simulink model "MPTC"  (R2023b)
settings: Solver=FixedStepDiscrete  StartTime=0.0  StopTime=0.4  RelTol=1e-3
model workspace (MAT data in the model file):
  Ts = 0.025
undefined symbols (not defined in the file): DiscIntNeverNeededParam
libraries: spsDCVoltageSourceLib x1, spsGroundLib x1, spsPermanentMagnetSynchronousMachineLib x1, slpidlib x1, spsThreePhaseVIMeasurementLib x1, spsUniversalBridgeLib x1, sps_lib x1
settings Model: Creator=rainy  LastModifiedBy=rainy

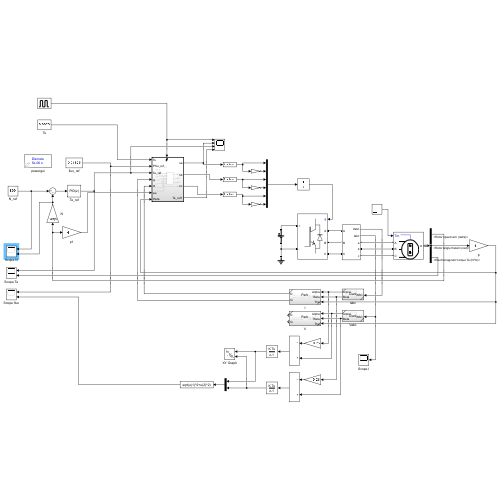
[thumbnail: Simulink's stored preview of the top-level diagram]
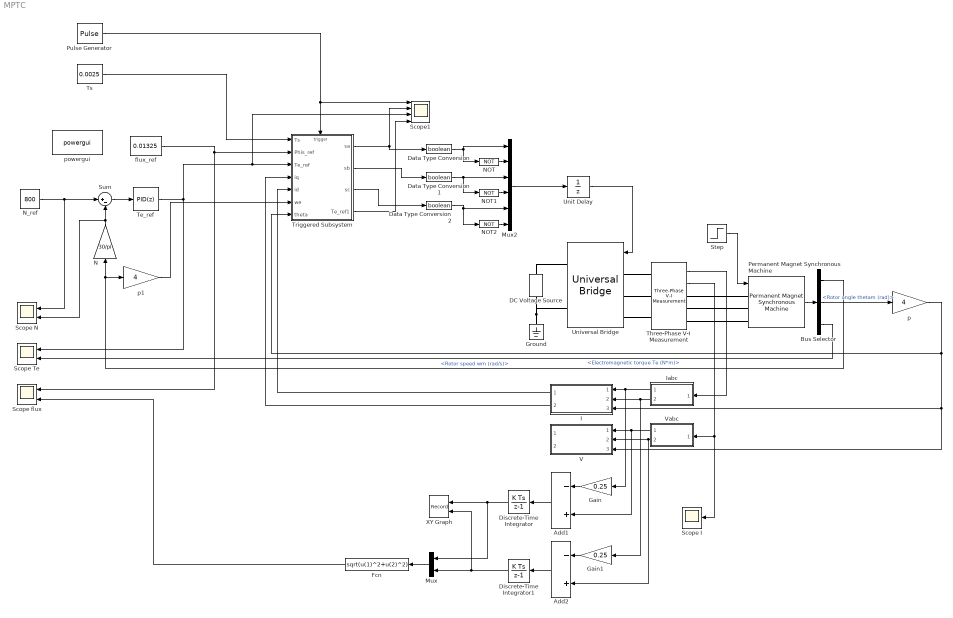
== system MPTC ==
  Add1 : Sum  Inputs=-+
  Add2 : Sum  Inputs=-+
  Bus Selector : BusSelector  OutputSignals=Rotor speed wm (rad/s),Rotor angle thetam (rad),Electromagnetic torque Te (N*m)
  DC Voltage Source : spsDCVoltageSourceLib/DC Voltage Source  Amplitude=24  Measurements=Voltage
  Data Type Conversion : DataTypeConversion  OutDataTypeStr=boolean  SaturateOnIntegerOverflow=off  RndMeth=Floor
  Data Type Conversion1 : DataTypeConversion  OutDataTypeStr=boolean  SaturateOnIntegerOverflow=off  RndMeth=Floor
  Data Type Conversion2 : DataTypeConversion  OutDataTypeStr=boolean  SaturateOnIntegerOverflow=off  RndMeth=Floor
  Discrete-Time Integrator : DiscreteIntegrator  SampleTime=-1  ICPrevOutput=DiscIntNeverNeededParam  ICPrevScaledInput=DiscIntNeverNeededParam
  Discrete-Time Integrator1 : DiscreteIntegrator  SampleTime=-1  ICPrevOutput=DiscIntNeverNeededParam  ICPrevScaledInput=DiscIntNeverNeededParam
  Fcn : Fcn  Expr=sqrt(u(1)^2+u(2)^2)
  Gain : Gain  Gain=0.25
  Gain1 : Gain  Gain=0.25
  Ground : spsGroundLib/Ground  LConnTagsString=a
  I : Subsystem  ReferencedSubsystem=Park
  Iabc : Subsystem  ReferencedSubsystem=Clark
  Mux : Mux  Inputs=2
  Mux2 : Mux  Inputs=6
  N : Gain  Gain=30/pi
  NOT : Logic  Operator=NOT  IconShape=distinctive  AllPortsSameDT=off  OutDataTypeStr=boolean
  NOT1 : Logic  Operator=NOT  IconShape=distinctive  AllPortsSameDT=off  OutDataTypeStr=boolean
  NOT2 : Logic  Operator=NOT  IconShape=distinctive  AllPortsSameDT=off  OutDataTypeStr=boolean
  N_ref : Constant  Value=800
  Permanent Magnet Synchronous Machine : spsPermanentMagnetSynchronousMachineLib/Permanent Magnet Synchronous Machine  NbPhases=3  FluxDistribution=Sinusoidal  RotorType=Round  MechanicalLoad=Torque Tm  PresetModel=No  ShowDetailedParameters=on  MeasurementBus=off  Resistance=0.25  Inductance=8.5e-3  dqInductances=[8.5e-3,8.5e-3]  La=0.0005  MachineConstant=Flux linkage established by magnets (V.s)  Flux=0.01325  VoltageCst=9.6131  TorqueCst=0.0795  Flat=120  Mechanical=[0.0008 0.0004924 4 0]  PolePairs=4  InitialConditions=[0,0, 0,0]  InitialConditions5ph=[0 0 0 0 0 0]  RefAngle=Aligned with phase A axis (original Park)  IterativeDiscreteModel=Trapezoidal non iterative  TsBlock=-1  TsPowergui=0
  Pulse Generator : DiscretePulseGenerator  PulseType=Time based  Period=0.0025
  Scope I : Scope
  Scope N : Scope  NumInputPorts=2
  Scope Te : Scope  NumInputPorts=2
  Scope flux : Scope  NumInputPorts=2
  Scope1 : Scope  NumInputPorts=4
  Step : Step  Time=0.2  SampleTime=0
  Sum : Sum  Inputs=|+-
  Te_ref : slpidlib/PID Controller  Controller=PID  Form=Parallel  TimeDomain=Discrete-time  UseExternalTs=off  SampleTime=-1  IntegratorMethod=Forward Euler  FilterMethod=Forward Euler  ControllerParametersSource=internal  P=2  I=1  UseKiTs=off  D=0  N=100  UseFilter=on  TunerSelectOption=Transfer Function Based (PID Tuner App)  InitialConditionSource=internal  InitialConditionForIntegrator=0  InitialConditionForFilter=0  DifferentiatorICPrevScaledInput=0  ExternalReset=none  TrackingMode=off  Kt=1  LimitOutput=off  SatLimitsSource=internal  UpperSaturationLimit=inf  LowerSaturationLimit=-inf  LinearizeAsGain=off  AntiWindupMode=none  Kb=1  LimitIntegrator=off  UpperIntegratorSaturationLimit=inf  LowerIntegratorSaturationLimit=-inf  POutMin=[]  POutMax=[]  IOutMin=[]  IOutMax=[]  DOutMin=[]  DOutMax=[]  NOutMin=[]  NOutMax=[]  SumOutMin=[]  SumOutMax=[]  SaturationOutMin=[]  SaturationOutMax=[]  PParamMin=[]  PParamMax=[]  IParamMin=[]  IParamMax=[]  DParamMin=[]  DParamMax=[]  NParamMin=[]  NParamMax=[]  KbParamMin=[]  KbParamMax=[]  KtParamMin=[]  KtParamMax=[]  KbOutMin=[]  KbOutMax=[]  KtOutMin=[]  KtOutMax=[]  IntegratorOutMin=[]  IntegratorOutMax=[]  FilterOutMin=[]  FilterOutMax=[]  SumI1OutMin=[]  SumI1OutMax=[]  SumI2OutMin=[]  SumI2OutMax=[]  SumI3OutMin=[]  SumI3OutMax=[]  SumI4OutMin=[]  SumI4OutMax=[]  SumDOutMin=[]  SumDOutMax=[]  DifferentiatorOutMin=[]  DifferentiatorOutMax=[]  FilterDiffOutCoefMin=[]  FilterDiffOutCoefMax=[]  ReciprocalOutMin=[]  ReciprocalOutMax=[]  SumDenOutMin=[]  SumDenOutMax=[]  SumNumOutMin=[]  SumNumOutMax=[]  DivideOutMin=[]  DivideOutMax=[]  UdiffTsProdOutMin=[]  UdiffTsProdOutMax=[]  NTsProdOutMin=[]  NTsProdOutMax=[]  UintegralTsProdOutMin=[]  UintegralTsProdOutMax=[]  UngainTsProdOutMin=[]  UngainTsProdOutMax=[]  ClampingZeroOutDataTypeStr=Inherit: Inherit via back propagation  ClampingZeroOutMin=[]  ClampingZeroOutMax=[]  FilterDenConstantOutDataTypeStr=Inherit: Inherit via back propagation  FilterDenConstantOutMin=[]  FilterDenConstantOutMax=[]  PCopyOutDataTypeStr=Inherit: Inherit via back propagation  PCopyOutMin=[]  PCopyOutMax=[]  NCopyOutDataTypeStr=Inherit: Inherit via back propagation  NCopyOutMin=[]  NCopyOutMax=[]  IntegratorContinuousStateAttributes=''  IntegratorStateMustResolveToSignalObject=off  IntegratorRTWStateStorageClass=Auto  FilterContinuousStateAttributes=''  FilterStateMustResolveToSignalObject=off  FilterRTWStateStorageClass=Auto  ParallelPVariant=InternalParameters  IdealPVariant=Disabled  IVariant=InternalParameters  DVariant=InternalParameters  IntegratorVariant=Discrete  SatVariant=Disabled  AWVariant=Passthrough  PCopyVariant=Disabled  TRVariant=Disabled  FdbkBlocksVariant=Forward  IdealPFdbkVariant=Disabled  SatFdbkVariant=Disabled  DerivativeFilterVariant=ForwardEulerFilter  NVariant=InternalParameters  NCopyVariant=Disabled  FilterICVariant=InternalICsFilter  IntegratorICVariant=InternalICs  ExternalResetVariant=Disabled  TRSumVariant=Passthrough  SumFdbkVariant=Disabled  SumVariant=Sum_PID  TsampFilterVariant=InternalTs  TsampNgainVariant=Passthrough  TsampIntegralVariant=Disabled_SignalSpec  ExternalSaturationOutDataTypeStr=Inherit: Same as second input
      settings: LibrarySourceBlock=simulink/Discrete/Discrete PID Controller
  Three-Phase V-I Measurement : spsThreePhaseVIMeasurementLib/Three-Phase V-I Measurement  VoltageMeasurement=phase-to-ground  SetLabelV=off  LabelV=Vabc  Vpu=off  VpuLL=off  CurrentMeasurement=yes  SetLabelI=off  LabelI=Iabc  Ipu=off  Pbase=100e6  Vbase=500e3  OutputType=Complex  PhasorSimulation=off  PSBequivalent=0
  Triggered Subsystem : Subsystem  TreatAsAtomicUnit=on
  Ts : Constant  Value=0.0025
  Unit Delay : UnitDelay  SampleTime=-1  HasFrameUpgradeWarning=on
  Universal Bridge : spsUniversalBridgeLib/Universal Bridge  Arms=3  SnubberResistance=1e5  SnubberCapacitance=inf  Device=IGBT / Diodes  Ron=1e-3  Lon=0  ForwardVoltages="[  0  0  ]"  ForwardVoltage=0  GTOparameters=[ 10e-6 , 20e-6 ]  IGBTparameters=[ 1e-6 , 2e-6 ]  Measurements=None  Measurements_2=None  converterType=Rectifier
  V : Subsystem  ReferencedSubsystem=Park
  Vabc : Subsystem  ReferencedSubsystem=Clark
  XY Graph : Record  FileSettingsInternal="{\"entries\":[{\"content\":{\"excelSettings\":{\"content\":{},\"type\":\"Streamout.ExcelSettings\"}},\"type\":\"Streamout.FileSettingStorage\",\"uuid\":\"\"}],\"packageUris\":[\"http:\\/\\/schema.mathworks.com\\/mf0\\/streamout_blocks\\/R2020a\"],\"version\":\"1.0\"}"  Layout=[1 1]  SignalsInternal="{\"entries\":[{\"content\":{\"signals\":[{\"content\":{\"blockPath\":[],\"dimensions\":[1],\"domain\":\"\",\"lineColor\":\"#a2142f\",\"plots\":[1],\"port\":1,\"sid\":[\"\"],\"signalID\":439,\"signalName\":\"Discrete-Time\\nIntegrator\"},\"type\":\"RecordBlkView.Signal\",\"uuid\":\"\"},{\"content\":{\"blockPath\":[],\"dimensions\":[1],\"domain\":\"\",\"lineColor\":\"#139fff\",\"plots\":[1],\"port\":2,\"sid\":[\"\"],\"signalID\":443,\"signalName\":\"Discrete-Time\\nIntegrator1\"},\"type\":\"RecordBlkView.Signal\",\"uuid\":\"\"}]},\"type\":\"RecordBlkView.InputSignals\",\"uuid\":\"\"}],\"packageUris\":[\"http:\\/\\/schema.mathworks.com\\/mf0\\/streamout_blocks\\/R2020a\"],\"version\":\"1.0\"}"  VisualizationBindings="{\"xyplotplugin\":{\"info\":[{\"series\":[{\"bindingParametersList\":[{\"parameter\":\"X-Axis\",\"signalID\":439,\"signalName\":\"Discrete-Time\\nIntegrator\"},{\"parameter\":\"Y-Axis\",\"signalID\":443,\"signalName\":\"Discrete-Time\\nIntegrator1\"}],\"seriesID\":125}],\"subplotID\":1}]}}"  CompatibilityTag=XY  st=-1
  flux_ref : Constant  Value=0.01325
  p : Gain  Gain=4
  p1 : Gain  Gain=4
  powergui : sps_lib/powergui  Priority=1  SimulationMode=Discrete  SampleTime=5e-6  frequency=60  Iterations=50  frequencyindice=0  Pbase=100e6  ErrMax=1e-4  UnitsV=kV  UnitsW=MW  buscounter=0  FunctionMessages=off  echomessages=off  EnableUseOfTLC=off  CurrentSourceSwitches=off  DisableSnubberDevices=off  DisableRonSwitches=off  DisableVfSwitches=off  DisplayEquations=off  AutomaticDiscreteSolvers=off  SolverType=Tustin/Backward Euler (TBE)  Interpol=off  ExternalGateDelay=off  methode=off  Ts=100  x0status=blocks  SPID=on  SwTol=0  HookPort=off  NonlinearTolerance=1e-4  nMaxIteration=100  ContinueOnMaxIteration=off  RestoreLinks=warning  ResistiveCurrentMeasurement=off  Frange=[0:2:500]  Ylog=off  Xlog=on  ShowGrid=off  save=off  variable=ZData  structure=0  ZoomFFT=off  StartTime=0.0  cycles=1  DisplayStyle=1  fundamental=60  FreqAxis=off  MaxFrequency=1000  frequencyindicesteady=1  RmsSteady=1  display=off
  wires:
  N_ref/1 -> Sum/1, Scope N/1
  Permanent Magnet Synchronous Machine/1 -> Bus Selector/1
  Bus Selector/1 -> p1/1, N/1  "<Rotor speed wm (rad/s)>"
  Three-Phase V-I Measurement/1 -> Iabc/1
  Three-Phase V-I Measurement/2 -> Scope I/1, Vabc/1
  Iabc/1 -> Gain/1, I/1
  Iabc/2 -> Gain1/1, I/2
  Unit Delay/1 -> Universal Bridge/1
  N/1 -> Sum/2, Scope N/2
  Sum/1 -> Te_ref/1
  flux_ref/1 -> Scope flux/1, Triggered Subsystem/2(Phis_ref)
  Te_ref/1 -> Scope1/3, Triggered Subsystem/3(Te_ref), Scope Te/1
  p/1 -> Triggered Subsystem/7(theta), I/3, V/3
  I/1 -> Triggered Subsystem/5(id)
  I/2 -> Triggered Subsystem/4(iq)
  p1/1 -> Triggered Subsystem/6(we)
  Step/1 -> Permanent Magnet Synchronous Machine/1
  Data Type Conversion/1 -> NOT/1, Mux2/1
  NOT1/1 -> Mux2/4
  NOT/1 -> Mux2/2
  NOT2/1 -> Mux2/6
  Data Type Conversion1/1 -> NOT1/1, Mux2/3
  Data Type Conversion2/1 -> NOT2/1, Mux2/5
  Triggered Subsystem/1(sa) -> Data Type Conversion/1, Scope1/2
  Triggered Subsystem/2(sb) -> Data Type Conversion1/1
  Triggered Subsystem/3(sc) -> Data Type Conversion2/1
  Mux2/1 -> Unit Delay/1
  Bus Selector/2 -> p/1  "<Rotor angle thetam (rad)>"
  Gain/1 -> Add1/1
  Vabc/1 -> Add1/2, V/1
  Vabc/2 -> Add2/2, V/2
  Gain1/1 -> Add2/1
  Add1/1 -> Discrete-Time Integrator/1
  Add2/1 -> Discrete-Time Integrator1/1
  Discrete-Time Integrator/1 -> Mux/1, XY Graph/1
  Discrete-Time Integrator1/1 -> XY Graph/2, Mux/2
  Bus Selector/3 -> Scope Te/2  "<Electromagnetic torque Te (N*m)>"
  Mux/1 -> Fcn/1
  Fcn/1 -> Scope flux/2
  Pulse Generator/1 -> Triggered Subsystem/Trigger, Scope1/1
  Ts/1 -> Triggered Subsystem/1(Ts)
  Triggered Subsystem/4(Te_ref1) -> Scope1/4
  connections:
  Ground/LConn1 -- Universal Bridge/RConn2 -- DC Voltage Source/LConn1
  Permanent Magnet Synchronous Machine/LConn2 -- Three-Phase V-I Measurement/RConn2
  Permanent Magnet Synchronous Machine/LConn1 -- Three-Phase V-I Measurement/RConn1
  Universal Bridge/LConn3 -- Three-Phase V-I Measurement/LConn3
  Universal Bridge/LConn1 -- Three-Phase V-I Measurement/LConn1
  Universal Bridge/LConn2 -- Three-Phase V-I Measurement/LConn2
  DC Voltage Source/RConn1 -- Universal Bridge/RConn1
  Permanent Magnet Synchronous Machine/LConn3 -- Three-Phase V-I Measurement/RConn3

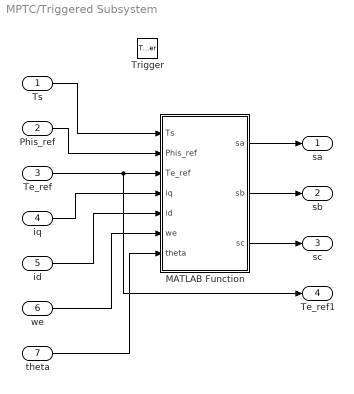
== system MPTC/Triggered Subsystem ==
  Ts : Inport
  Phis_ref : Inport  Port=2
  Te_ref : Inport  Port=3
  iq : Inport  Port=4
  id : Inport  Port=5
  we : Inport  Port=6
  theta : Inport  Port=7
  Trigger : TriggerPort  VariantControl=(inherit)
  MATLAB Function : MATLAB Function  TreatAsAtomicUnit=on
  sa : Outport
  sb : Outport  Port=2
  sc : Outport  Port=3
  Te_ref1 : Outport  Port=4
  wires:
  Phis_ref/1 -> MATLAB Function/2(Phis_ref)
  Te_ref/1 -> Te_ref1/1, MATLAB Function/3(Te_ref)
  iq/1 -> MATLAB Function/4(iq)
  id/1 -> MATLAB Function/5(id)
  we/1 -> MATLAB Function/6(we)
  theta/1 -> MATLAB Function/7(theta)
  MATLAB Function/1(sa) -> sa/1
  MATLAB Function/2(sb) -> sb/1
  MATLAB Function/3(sc) -> sc/1
  Ts/1 -> MATLAB Function/1(Ts)

== matlab function MPTC/Triggered Subsystem/MATLAB Function ==
  data: Ts input; Phis_ref input; sa output; Te_ref input; iq input; id input; we input; theta input; sb output; sc output
function [sa, sb, sc] = fcn(Ts, Phis_ref, Te_ref, iq, id, we, theta)

R       = 0.25;
Ld      = 0.0005;
Lq      = 0.0005;
Phif    = 0.01325;
p       = 4;
Vdc     = 24;
gmin    = 20000000;
m       = 50;
imin    = 1;

sw = [0 0 0; 0 0 1; 0 1 0; 0 1 1; 1 0 0; 1 0 1; 1 1 0; 1 1 1];
trans = 2/3*[cos(theta) cos(theta-2/3*pi) cos(theta+2/3*pi);
             -sin(theta) -sin(theta-2/3*pi) -sin(theta+2/3*pi)];

persistent flag ud_prev uq_prev ud_next uq_next
if isempty(flag)
    flag = 1;
    ud_prev = 0;
    uq_prev = 0;
    ud_next = 0;
    uq_next = 0;
end

ud_prev = ud_next;
uq_prev = uq_next;

id1 = id+Ts/Ld*(ud_prev+iq*we*Lq-id*R);
iq1 = iq+Ts/Lq*(uq_prev-id*we*Ld-iq*R-Phif*we);
for i=1:8
    sa = sw(i,1); sb = sw(i, 2); sc = sw(i, 3);
    Va = Vdc*(2*sa-sb-sc)/3;
    Vb = Vdc*(2*sb-sc-sa)/3;
    Vc = Vdc*(2*sc-sa-sb)/3;
    Vabc = [Va; Vb; Vc];
    Vdq = trans*Vabc;
    Vd = Vdq(1, 1);
    Vq = Vdq(2, 1);
    id2 = id1+Ts/Ld*(Vd+iq1*we*Lq-id1*R);
    iq2 = iq1+Ts/Lq*(Vq-id1*we*Ld-iq1*R-Phif*we);
    Te2 = 3/2*p*iq2*Phif;
    Phid2 = Ld*id2+Phif;
    Phiq2 = Lq*iq2;
    Phis2 = (Phid2^2+Phiq2^2)^0.5;
    d_Te = abs(Te_ref - Te2);
    d_Phis = abs(Phis_ref-Phis2);
    g = abs(Te_ref - Te2)+m*abs(Phis_ref-Phis2);
    [i g d_Te m*d_Phis];
    if (g<gmin)
        imin = i;
        gmin = g;
    end
end

sa = sw(imin,1); sb = sw(imin, 2); sc = sw(imin, 3);
Va = Vdc*(2*sa-sb-sc)/3;
Vb = Vdc*(2*sb-sc-sa)/3;
Vc = Vdc*(2*sc-sa-sb)/3;
Vabc = [Va; Vb; Vc];
Vdq = trans*Vabc;
ud_next = Vdq(1, 1);
uq_next = Vdq(2, 1);
